simulink model "Microgrid"  (R2020b)
settings: Solver=VariableStepAuto  StartTime=0.0  StopTime=5  RelTol=1e-3
libraries: dspstat3 x1
settings Model: Creator=Stefano  LastModifiedBy=stefanopanzieri
settings SFSimCC: CustomCodeUndefinedFunction=UseInterfaceOnly

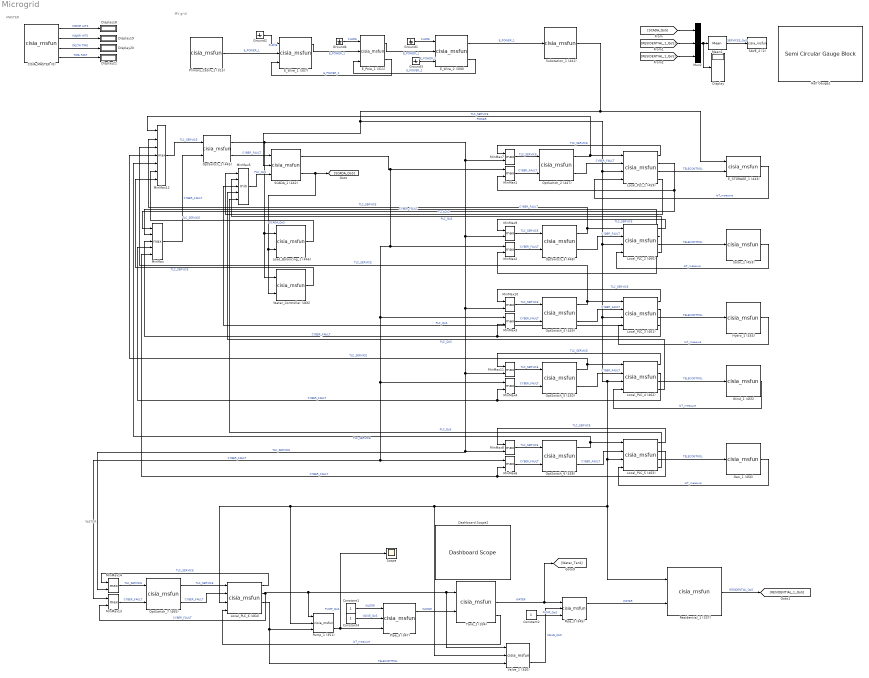
== system Microgrid ==
  note: MV grid
  note: MASTER
  note: WATER
  CISIA_MASTER (0) : M-S-Function  FunctionName=cisia_msfun  Parameters=Parameter1, Parameter2, Parameter3, resources, Parameter4, Parameter5, Parameter6, Parameter7, Parameter8, Parameter9  mask(S-function:msfcn_unit_delay){Parameter1='CISIA_MASTER', Parameter2=0.001, Parameter3='SistemiIoT', resources=off, Parameter4=on, Parameter5=off, Parameter6=off, Parameter7=off, Parameter8=1, Parameter9=off}
      mask prompts: Parameter1 "entity name"; Parameter2 "sampling time"; Parameter3 "project"; resources "Save status at each major hit"; Parameter4 "Show Operative Levels with colors"; Parameter5 "Load Entities from file"; Parameter6 "Load Start from Mask"; Parameter7 "Real Time"; Parameter8 "Real Time Hit (sec)"; Parameter9 "Skip saving"
      mask help: This is a level-2 MATLAB file S-function which demonstrates CISIA entity
      mask Display: disp('MASTER BLOCK')
  Constant1 : Constant
  Constant2 : Constant
  Constant4 : Constant
  Dashboard Scope2 : DashboardScope  Ymin=0  Ymax=1
  Display{,18..21} (5 alike) : Display
  E_Pole_1 (311) : M-S-Function  FunctionName=cisia_msfun  Parameters=Parameter1, Parameter2, Parameter3, resources, Parameter10, codeupdate, step_received, step_computed, dynamic_computed, step_sended, id_entity, id_project, id_type, name_type, color  mask(S-function:msfcn_unit_delay){Parameter1='E_Pole_1', Parameter2=1, Parameter3='', resources=|, Parameter10=off, codeupdate=off, step_received=|, step_computed=, dynamic_computed=, step_sended=|, id_entity=311, id_project=6, id_type=68, name_type=Electric_Pole, color=#FFFFFF}
      mask resources=|
      | *** INPUT RESOURCES ***
      | NUM_INPUTS 3
      | FLAME (1)
      | E_POWER_1 (10)
      | E_POWER_2 (10)
      |
      | *** STATE VARIABLES ***
      | NUM_VARIABLES 5
      | Operative_Level(NUMERIC)(1)(1)
      | Mechanical_Fault(NUMERIC)(1)(0)
      | Fire_Fault(NUMERIC)(1)(0)
      | Physical_Fault(NUMERIC)(1)(0)
      | Power_Gen(NUMERIC_ARRAY)(10)(0  0  0  0  0  0  0  0  0  0)
      |
      | *** OUTPUT RESOURCES ***
      | NUM_OUTPUTS 2
      | E_POWER_1 (10)
      | E_POWER_2 (10)
      mask step_received=|
      | Power_Gen=max(E_POWER_1,E_POWER_2);
      |
      | Fire_Fault=FLAME;
      |
      | Physical_Fault=max(Fire_Fault,Mechanical_Fault);
      |
      | Operative_Level=1-Physical_Fault;
      mask step_sended=|
      | E_POWER_1=Power_Gen*(1-Physical_Fault);
      | E_POWER_2=Power_Gen*(1-Physical_Fault);
      mask prompts: Parameter1 "entity name"; Parameter2 "sampling time"; Parameter3 "project"; resources "input resources and state variables"; Parameter10 "Bring state variables to output"; codeupdate "update code from mask"
      mask help: This is a level-2 MATLAB file S-function which demonstrates CISIA entity
      mask DialogControl Container1 Prompt: All parameters
      mask Display: image('Icons/Electric_Pole.png')
  E_STORAGE_1 (443) : M-S-Function  FunctionName=cisia_msfun  Parameters=Parameter1, Parameter2, Parameter3, resources, Parameter10, codeupdate, step_received, step_computed, dynamic_computed, step_sended, id_entity, id_project, id_type, name_type, color  mask(S-function:msfcn_unit_delay){Parameter1='E_STORAGE_1', Parameter2=1, Parameter3='', resources=|, Parameter10=off, codeupdate=off, step_received=|, step_computed=, dynamic_computed=, step_sended=IoT_measure=(1-IoT_Fault)*Operative_Level;, id_entity=443, id_project=6, id_type=101, name_type=Energy_Storage, color=#FFFFFF}
      mask resources=|
      | *** INPUT RESOURCES ***
      | NUM_INPUTS 2
      | POWER (1)
      | TELECONTROL (1)
      |
      | *** STATE VARIABLES ***
      | NUM_VARIABLES 5
      | Operative_Level(NUMERIC)(1)(1)
      | Cyber_Fault(NUMERIC_ARRAY)(10)(0  0  0  0  0  0  0  0  0  0)
      | Mechanical_Fault(NUMERIC)(1)(0)
      | Control_Fault(NUMERIC)(1)(0)
      | IoT_Fault(NUMERIC)(1)(0)
      |
      | *** OUTPUT RESOURCES ***
      | NUM_OUTPUTS 1
      | IoT_measure (1)
      mask step_received=|
      | Control_Fault=max([1-TELECONTROL Mechanical_Fault]);
      |
      | Operative_Level=min([1- Control_Fault 1-Mechanical_Fault POWER]);
      mask prompts: Parameter1 "entity name"; Parameter2 "sampling time"; Parameter3 "project"; resources "input resources and state variables"; Parameter10 "Bring state variables to output"; codeupdate "update code from mask"
      mask help: This is a level-2 MATLAB file S-function which demonstrates CISIA entity
      mask DialogControl Container1 Prompt: All parameters
      mask Display: image('Icons/Energy_Storage.png')
  E_Wire_1 (307) : M-S-Function  FunctionName=cisia_msfun  Parameters=Parameter1, Parameter2, Parameter3, resources, Parameter10, codeupdate, step_received, step_computed, dynamic_computed, step_sended, id_entity, id_project, id_type, name_type, color  mask(S-function:msfcn_unit_delay){Parameter1='E_Wire_1', Parameter2=1, Parameter3='', resources=|, Parameter10=off, codeupdate=off, step_received=|, step_computed=, dynamic_computed=, step_sended=|, id_entity=307, id_project=6, id_type=67, name_type=Electric_Wire, color=#FFFFFF}
      mask resources=|
      | *** INPUT RESOURCES ***
      | NUM_INPUTS 3
      | FLAME (1)
      | E_POWER_1 (10)
      | E_POWER_2 (10)
      |
      | *** STATE VARIABLES ***
      | NUM_VARIABLES 5
      | Operative_Level(NUMERIC)(1)(1)
      | Mechanical_Fault(NUMERIC)(1)(0)
      | Fire_Fault(NUMERIC)(1)(0)
      | Physical_Fault(NUMERIC)(1)(0)
      | Power_Gen(NUMERIC_ARRAY)(10)(0  0  0  0  0  0  0  0  0  0)
      |
      | *** OUTPUT RESOURCES ***
      | NUM_OUTPUTS 2
      | E_POWER_1 (10)
      | E_POWER_2 (10)
      mask step_received=|
      | Power_Gen=max(E_POWER_1,E_POWER_2);
      |
      | Fire_Fault=FLAME;
      |
      | Physical_Fault=max(Fire_Fault,Mechanical_Fault);
      |
      | Operative_Level=1-Physical_Fault;
      mask step_sended=|
      | E_POWER_1=Power_Gen*(1-Physical_Fault);
      | E_POWER_2=Power_Gen*(1-Physical_Fault);
      mask prompts: Parameter1 "entity name"; Parameter2 "sampling time"; Parameter3 "project"; resources "input resources and state variables"; Parameter10 "Bring state variables to output"; codeupdate "update code from mask"
      mask help: This is a level-2 MATLAB file S-function which demonstrates CISIA entity
      mask DialogControl Container1 Prompt: All parameters
      mask Display: image('Icons/Electric_Wire.png')
  E_Wire_2 (308) : M-S-Function  FunctionName=cisia_msfun  Parameters=Parameter1, Parameter2, Parameter3, resources, Parameter10, codeupdate, step_received, step_computed, dynamic_computed, step_sended, id_entity, id_project, id_type, name_type, color  mask(S-function:msfcn_unit_delay){Parameter1='E_Wire_2', Parameter2=1, Parameter3='', resources=|, Parameter10=off, codeupdate=off, step_received=|, step_computed=, dynamic_computed=, step_sended=|, id_entity=308, id_project=6, id_type=67, name_type=Electric_Wire, color=#FFFFFF}
      mask resources=|
      | *** INPUT RESOURCES ***
      | NUM_INPUTS 3
      | FLAME (1)
      | E_POWER_1 (10)
      | E_POWER_2 (10)
      |
      | *** STATE VARIABLES ***
      | NUM_VARIABLES 5
      | Operative_Level(NUMERIC)(1)(1)
      | Mechanical_Fault(NUMERIC)(1)(0)
      | Fire_Fault(NUMERIC)(1)(0)
      | Physical_Fault(NUMERIC)(1)(0)
      | Power_Gen(NUMERIC_ARRAY)(10)(0  0  0  0  0  0  0  0  0  0)
      |
      | *** OUTPUT RESOURCES ***
      | NUM_OUTPUTS 2
      | E_POWER_1 (10)
      | E_POWER_2 (10)
      mask step_received=|
      | Power_Gen=max(E_POWER_1,E_POWER_2);
      |
      | Fire_Fault=FLAME;
      |
      | Physical_Fault=max(Fire_Fault,Mechanical_Fault);
      |
      | Operative_Level=1-Physical_Fault;
      mask step_sended=|
      | E_POWER_1=Power_Gen*(1-Physical_Fault);
      | E_POWER_2=Power_Gen*(1-Physical_Fault);
      mask prompts: Parameter1 "entity name"; Parameter2 "sampling time"; Parameter3 "project"; resources "input resources and state variables"; Parameter10 "Bring state variables to output"; codeupdate "update code from mask"
      mask help: This is a level-2 MATLAB file S-function which demonstrates CISIA entity
      mask DialogControl Container1 Prompt: All parameters
      mask Display: image('Icons/Electric_Wire.png')
  Geo_1 (456) : M-S-Function  FunctionName=cisia_msfun  Parameters=Parameter1, Parameter2, Parameter3, resources, Parameter10, codeupdate, step_received, step_computed, dynamic_computed, step_sended, id_entity, id_project, id_type, name_type, color  mask(S-function:msfcn_unit_delay){Parameter1='Geo_1', Parameter2=1, Parameter3='', resources=|, Parameter10=off, codeupdate=off, step_received=|, step_computed=, dynamic_computed=, step_sended=IoT_measure=(1-IoT_Fault)*Operative_Level;, id_entity=456, id_project=6, id_type=107, name_type=Geothermic, color=#FFFFFF}
      mask resources=|
      | *** INPUT RESOURCES ***
      | NUM_INPUTS 1
      | TELECONTROL (1)
      |
      | *** STATE VARIABLES ***
      | NUM_VARIABLES 5
      | Operative_Level(NUMERIC)(1)(1)
      | Mechanical_Fault(NUMERIC)(1)(0)
      | Consumed_Services(NUMERIC_ARRAY)(20)(1  0  0  0  0  0  0  0  0  0  0  0  0  0  0  0  0  0  0  0)
      | Control_Fault(NUMERIC)(1)(0)
      | IoT_Fault(NUMERIC)(1)(0)
      |
      | *** OUTPUT RESOURCES ***
      | NUM_OUTPUTS 1
      | IoT_measure (1)
      mask step_received=|
      | Control_Fault=max([1-TELECONTROL Mechanical_Fault]);
      |
      | Operative_Level=min([1- Control_Fault 1-Mechanical_Fault]);
      mask prompts: Parameter1 "entity name"; Parameter2 "sampling time"; Parameter3 "project"; resources "input resources and state variables"; Parameter10 "Bring state variables to output"; codeupdate "update code from mask"
      mask help: This is a level-2 MATLAB file S-function which demonstrates CISIA entity
      mask DialogControl Container1 Prompt: All parameters
      mask Display: image('Icons/Geothermic.png')
  Ground{1..4} (4 alike) : Ground
  Half Gauge1 : SemiCircularGaugeBlock  ScaleMax=1
  Hydro_1 (454) : M-S-Function  FunctionName=cisia_msfun  Parameters=Parameter1, Parameter2, Parameter3, resources, Parameter10, codeupdate, step_received, step_computed, dynamic_computed, step_sended, id_entity, id_project, id_type, name_type, color  mask(S-function:msfcn_unit_delay){Parameter1='Hydro_1', Parameter2=1, Parameter3='', resources=|, Parameter10=off, codeupdate=off, step_received=|, step_computed=, dynamic_computed=, step_sended=IoT_measure=(1-IoT_Fault)*Operative_Level;, id_entity=454, id_project=6, id_type=105, name_type=Hydroelectric, color=#FFFFFF}
      mask resources=|
      | *** INPUT RESOURCES ***
      | NUM_INPUTS 1
      | TELECONTROL (1)
      |
      | *** STATE VARIABLES ***
      | NUM_VARIABLES 5
      | Operative_Level(NUMERIC)(1)(1)
      | Mechanical_Fault(NUMERIC)(1)(0)
      | Consumed_Services(NUMERIC_ARRAY)(20)(1  0  0  0  0  0  0  0  0  0  0  0  0  0  0  0  0  0  0  0)
      | Control_Fault(NUMERIC)(1)(0)
      | IoT_Fault(NUMERIC)(1)(0)
      |
      | *** OUTPUT RESOURCES ***
      | NUM_OUTPUTS 1
      | IoT_measure (1)
      mask step_received=|
      | Control_Fault=max([1-TELECONTROL Mechanical_Fault]);
      |
      | Operative_Level=min([1- Control_Fault 1-Mechanical_Fault]);
      mask prompts: Parameter1 "entity name"; Parameter2 "sampling time"; Parameter3 "project"; resources "input resources and state variables"; Parameter10 "Bring state variables to output"; codeupdate "update code from mask"
      mask help: This is a level-2 MATLAB file S-function which demonstrates CISIA entity
      mask DialogControl Container1 Prompt: All parameters
      mask Display: image('Icons/Hydroelectric.png')
  Load_Balancing_1 (446) : M-S-Function  FunctionName=cisia_msfun  Parameters=Parameter1, Parameter2, Parameter3, resources, Parameter10, codeupdate, step_received, step_computed, dynamic_computed, step_sended, id_entity, id_project, id_type, name_type, color  mask(S-function:msfcn_unit_delay){Parameter1='Load_Balancing_1', Parameter2=1, Parameter3='', resources=|, Parameter10=off, codeupdate=off, step_received=|, step_computed=, dynamic_computed=, step_sended=TLC_SERVICE=TLC_services*(1-Mechanical_Fault);, id_entity=446, id_project=6, id_type=103, name_type=Intelligent_Controller, color=#FFFFFF}
      mask resources=|
      | *** INPUT RESOURCES ***
      | NUM_INPUTS 2
      | TLC_SERVICE (20)
      | SCADA_QoS (1)
      |
      | *** STATE VARIABLES ***
      | NUM_VARIABLES 5
      | Operative_Level(NUMERIC)(1)(1)
      | TLC_services(NUMERIC_ARRAY)(20)(1  0  0  0  0  0  0  0  0  0  0  0  0  0  0  0  0  0  0  0)
      | Mechanical_Fault(NUMERIC)(1)(0)
      | Consumed_Services(NUMERIC_ARRAY)(20)(0  1  1  1  1  1  0  0  0  0  0  0  0  0  0  0  0  0  0  0)
      | Service_Fault(NUMERIC)(1)(0)
      |
      | *** OUTPUT RESOURCES ***
      | NUM_OUTPUTS 1
      | TLC_SERVICE (20)
      mask step_received=|
      | TLC_services=max(TLC_services_init,TLC_SERVICE);
      |
      | Service_Fault=max(abs(Consumed_Services.*TLC_services-Consumed_Services));
      |
      | Operative_Level=min([1-Mechanical_Fault 1-Service_Fault]);
      mask prompts: Parameter1 "entity name"; Parameter2 "sampling time"; Parameter3 "project"; resources "input resources and state variables"; Parameter10 "Bring state variables to output"; codeupdate "update code from mask"
      mask help: This is a level-2 MATLAB file S-function which demonstrates CISIA entity
      mask DialogControl Container1 Prompt: All parameters
      mask Display: image('Icons/Intelligent_Controller.png')
  Local_PLC_1 (459) : M-S-Function  FunctionName=cisia_msfun  Parameters=Parameter1, Parameter2, Parameter3, resources, Parameter10, codeupdate, step_received, step_computed, dynamic_computed, step_sended, id_entity, id_project, id_type, name_type, color  mask(S-function:msfcn_unit_delay){Parameter1='Local_PLC_1', Parameter2=1, Parameter3='', resources=|, Parameter10=off, codeupdate=off, step_received=|, step_computed=, dynamic_computed=, step_sended=|, id_entity=459, id_project=6, id_type=108, name_type=LocalController, color=#FFFFFF}
      mask resources=|
      | *** INPUT RESOURCES ***
      | NUM_INPUTS 4
      | TLC_SERVICE (20)
      | CYBER_FAULT (10)
      | POWER (1)
      | IoT_measure (1)
      |
      | *** STATE VARIABLES ***
      | NUM_VARIABLES 17
      | Operative_Level(NUMERIC)(1)(1)
      | TLC_services(NUMERIC_ARRAY)(20)(0  1  0  0  0  0  0  0  0  0  0  0  0  0  0  0  0  0  0  0)
      | Dos_attack(NUMERIC)(1)(0)
      | MITM_attack(NUMERIC)(1)(0)
      | Virus_Attack(NUMERIC)(1)(0)
      | Port_Scan_Attack(NUMERIC)(1)(0)
      | Cyber_Fault(NUMERIC_ARRAY)(10)(0  0  0  0  0  0  0  0  0  0)
      | BGP_hijacking(NUMERIC)(1)(0)
      | Mechanical_Fault(NUMERIC)(1)(0)
      | Consumed_Services(NUMERIC_ARRAY)(20)(1  0  0  0  0  0  0  0  0  0  0  0  0  0  0  0  0  0  0  0)
      | Service_Fault(NUMERIC)(1)(0)
      | BotNet_Attack(NUMERIC)(1)(0)
      | Data_Corruption(NUMERIC)(1)(0)
      | SW_Change(NUMERIC)(1)(0)
      | Config_Change(NUMERIC)(1)(0)
      | Port_Saturation(NUMERIC)(1)(0)
      | Control_Fault(NUMERIC)(1)(0)
      |
      | *** OUTPUT RESOURCES ***
      | NUM_OUTPUTS 4
      | TLC_SERVICE (20)
      | CYBER_FAULT (10)
      | TELECONTROL (1)
      | PLC_QoS (1)
      mask step_received=|
      | TLC_services=max(TLC_services_init,TLC_SERVICE);
      |
      | Service_Fault=max(abs(Consumed_Services.*TLC_services-Consumed_Services));
      |
      | Cyber_Fault=max(CYBER_FAULT, transpose([Dos_attack MITM_attack Virus_Attack Port_Scan_Attack  BGP_hijacking BotNet_Attack Data_Corruption SW_Change Config_Change Port_Saturation]));
      |
      |
      | %Control_Fault=max([1-Service_Fault Mechanical_Fault 1-POWER Dos_attack min(0.5,max(Cyber_Fault))]);
      |
      | Control_Fault=max([Service_Fault Mechanical_Fault 1-POWER Dos_attack min(0.5,max(Cyber_Fault))]);
      |
      |
      | Operative_Level=min([1-max(Cyber_Fault) 1-Mechanical_Fault 1-Control_Fault 1-Service_Fault]);
      mask step_sended=|
      | CYBER_FAULT=Cyber_Fault.*transpose([0 0 0.5 0.2 0 0 0 0 0 0]);
      |
      | TELECONTROL=1-Control_Fault;
      | PLC_QoS=Operative_Level;
      |
      | TLC_SERVICE=TLC_services;
      mask prompts: Parameter1 "entity name"; Parameter2 "sampling time"; Parameter3 "project"; resources "input resources and state variables"; Parameter10 "Bring state variables to output"; codeupdate "update code from mask"
      mask help: This is a level-2 MATLAB file S-function which demonstrates CISIA entity
      mask DialogControl Container1 Prompt: All parameters
      mask Display: image('Icons/LocalController.png')
  Local_PLC_2 (460) : M-S-Function  FunctionName=cisia_msfun  Parameters=Parameter1, Parameter2, Parameter3, resources, Parameter10, codeupdate, step_received, step_computed, dynamic_computed, step_sended, id_entity, id_project, id_type, name_type, color  mask(S-function:msfcn_unit_delay){Parameter1='Local_PLC_2', Parameter2=1, Parameter3='', resources=|, Parameter10=off, codeupdate=off, step_received=|, step_computed=, dynamic_computed=, step_sended=|, id_entity=460, id_project=6, id_type=108, name_type=LocalController, color=#FFFFFF}
      mask resources=|
      | *** INPUT RESOURCES ***
      | NUM_INPUTS 4
      | TLC_SERVICE (20)
      | CYBER_FAULT (10)
      | POWER (1)
      | IoT_measure (1)
      |
      | *** STATE VARIABLES ***
      | NUM_VARIABLES 17
      | Operative_Level(NUMERIC)(1)(0)
      | TLC_services(NUMERIC_ARRAY)(20)(0  0  1  0  0  0  0  0  0  0  0  0  0  0  0  0  0  0  0  0)
      | Dos_attack(NUMERIC)(1)(0.5)
      | MITM_attack(NUMERIC)(1)(0)
      | Virus_Attack(NUMERIC)(1)(0)
      | Port_Scan_Attack(NUMERIC)(1)(0)
      | Cyber_Fault(NUMERIC_ARRAY)(10)(0  0  0  0  0  0  0  0  0  0)
      | BGP_hijacking(NUMERIC)(1)(0)
      | Mechanical_Fault(NUMERIC)(1)(0)
      | Consumed_Services(NUMERIC_ARRAY)(20)(1  0  0  0  0  0  0  0  0  0  0  0  0  0  0  0  0  0  0  0)
      | Service_Fault(NUMERIC)(1)(0)
      | BotNet_Attack(NUMERIC)(1)(0)
      | Data_Corruption(NUMERIC)(1)(0)
      | SW_Change(NUMERIC)(1)(0)
      | Config_Change(NUMERIC)(1)(0)
      | Port_Saturation(NUMERIC)(1)(0)
      | Control_Fault(NUMERIC)(1)(0)
      |
      | *** OUTPUT RESOURCES ***
      | NUM_OUTPUTS 4
      | TLC_SERVICE (20)
      | CYBER_FAULT (10)
      | TELECONTROL (1)
      | PLC_QoS (1)
      mask step_received=|
      | TLC_services=max(TLC_services_init,TLC_SERVICE);
      |
      | Service_Fault=max(abs(Consumed_Services.*TLC_services-Consumed_Services));
      |
      | Cyber_Fault=max(CYBER_FAULT, transpose([Dos_attack MITM_attack Virus_Attack Port_Scan_Attack  BGP_hijacking BotNet_Attack Data_Corruption SW_Change Config_Change Port_Saturation]));
      |
      |
      | %Control_Fault=max([1-Service_Fault Mechanical_Fault 1-POWER Dos_attack min(0.5,max(Cyber_Fault))]);
      |
      | Control_Fault=max([Service_Fault Mechanical_Fault 1-POWER Dos_attack min(0.5,max(Cyber_Fault))]);
      |
      |
      | Operative_Level=min([1-max(Cyber_Fault) 1-Mechanical_Fault 1-Control_Fault 1-Service_Fault]);
      mask step_sended=|
      | CYBER_FAULT=Cyber_Fault.*transpose([0 0 0.5 0.2 0 0 0 0 0 0]);
      |
      | TELECONTROL=1-Control_Fault;
      | PLC_QoS=Operative_Level;
      |
      | TLC_SERVICE=TLC_services;
      mask prompts: Parameter1 "entity name"; Parameter2 "sampling time"; Parameter3 "project"; resources "input resources and state variables"; Parameter10 "Bring state variables to output"; codeupdate "update code from mask"
      mask help: This is a level-2 MATLAB file S-function which demonstrates CISIA entity
      mask DialogControl Container1 Prompt: All parameters
      mask Display: image('Icons/LocalController.png')
  Local_PLC_3 (461) : M-S-Function  FunctionName=cisia_msfun  Parameters=Parameter1, Parameter2, Parameter3, resources, Parameter10, codeupdate, step_received, step_computed, dynamic_computed, step_sended, id_entity, id_project, id_type, name_type, color  mask(S-function:msfcn_unit_delay){Parameter1='Local_PLC_3', Parameter2=1, Parameter3='', resources=|, Parameter10=off, codeupdate=off, step_received=|, step_computed=, dynamic_computed=, step_sended=|, id_entity=461, id_project=6, id_type=108, name_type=LocalController, color=#FFFFFF}
      mask resources=|
      | *** INPUT RESOURCES ***
      | NUM_INPUTS 4
      | TLC_SERVICE (20)
      | CYBER_FAULT (10)
      | POWER (1)
      | IoT_measure (1)
      |
      | *** STATE VARIABLES ***
      | NUM_VARIABLES 17
      | Operative_Level(NUMERIC)(1)(0)
      | TLC_services(NUMERIC_ARRAY)(20)(0  0  0  1  0  0  0  0  0  0  0  0  0  0  0  0  0  0  0  0)
      | Dos_attack(NUMERIC)(1)(0)
      | MITM_attack(NUMERIC)(1)(0)
      | Virus_Attack(NUMERIC)(1)(0)
      | Port_Scan_Attack(NUMERIC)(1)(0)
      | Cyber_Fault(NUMERIC_ARRAY)(10)(0  0  0  0  0  0  0  0  0  0)
      | BGP_hijacking(NUMERIC)(1)(0)
      | Mechanical_Fault(NUMERIC)(1)(0)
      | Consumed_Services(NUMERIC_ARRAY)(20)(1  0  0  0  0  0  0  0  0  0  0  0  0  0  0  0  0  0  0  0)
      | Service_Fault(NUMERIC)(1)(0)
      | BotNet_Attack(NUMERIC)(1)(0)
      | Data_Corruption(NUMERIC)(1)(0)
      | SW_Change(NUMERIC)(1)(0)
      | Config_Change(NUMERIC)(1)(0)
      | Port_Saturation(NUMERIC)(1)(0)
      | Control_Fault(NUMERIC)(1)(0)
      |
      | *** OUTPUT RESOURCES ***
      | NUM_OUTPUTS 4
      | TLC_SERVICE (20)
      | CYBER_FAULT (10)
      | TELECONTROL (1)
      | PLC_QoS (1)
      mask step_received=|
      | TLC_services=max(TLC_services_init,TLC_SERVICE);
      |
      | Service_Fault=max(abs(Consumed_Services.*TLC_services-Consumed_Services));
      |
      | Cyber_Fault=max(CYBER_FAULT, transpose([Dos_attack MITM_attack Virus_Attack Port_Scan_Attack  BGP_hijacking BotNet_Attack Data_Corruption SW_Change Config_Change Port_Saturation]));
      |
      |
      | %Control_Fault=max([1-Service_Fault Mechanical_Fault 1-POWER Dos_attack min(0.5,max(Cyber_Fault))]);
      |
      | Control_Fault=max([Service_Fault Mechanical_Fault 1-POWER Dos_attack min(0.5,max(Cyber_Fault))]);
      |
      |
      | Operative_Level=min([1-max(Cyber_Fault) 1-Mechanical_Fault 1-Control_Fault 1-Service_Fault]);
      mask step_sended=|
      | CYBER_FAULT=Cyber_Fault.*transpose([0 0 0.5 0.2 0 0 0 0 0 0]);
      |
      | TELECONTROL=1-Control_Fault;
      | PLC_QoS=Operative_Level;
      |
      | TLC_SERVICE=TLC_services;
      mask prompts: Parameter1 "entity name"; Parameter2 "sampling time"; Parameter3 "project"; resources "input resources and state variables"; Parameter10 "Bring state variables to output"; codeupdate "update code from mask"
      mask help: This is a level-2 MATLAB file S-function which demonstrates CISIA entity
      mask DialogControl Container1 Prompt: All parameters
      mask Display: image('Icons/LocalController.png')
  Local_PLC_4 (462) : M-S-Function  FunctionName=cisia_msfun  Parameters=Parameter1, Parameter2, Parameter3, resources, Parameter10, codeupdate, step_received, step_computed, dynamic_computed, step_sended, id_entity, id_project, id_type, name_type, color  mask(S-function:msfcn_unit_delay){Parameter1='Local_PLC_4', Parameter2=1, Parameter3='', resources=|, Parameter10=off, codeupdate=off, step_received=|, step_computed=, dynamic_computed=, step_sended=|, id_entity=462, id_project=6, id_type=108, name_type=LocalController, color=#FFFFFF}
      mask resources=|
      | *** INPUT RESOURCES ***
      | NUM_INPUTS 4
      | TLC_SERVICE (20)
      | CYBER_FAULT (10)
      | POWER (1)
      | IoT_measure (1)
      |
      | *** STATE VARIABLES ***
      | NUM_VARIABLES 17
      | Operative_Level(NUMERIC)(1)(0)
      | TLC_services(NUMERIC_ARRAY)(20)(0  0  0  0  1  0  0  0  0  0  0  0  0  0  0  0  0  0  0  0)
      | Dos_attack(NUMERIC)(1)(0)
      | MITM_attack(NUMERIC)(1)(0)
      | Virus_Attack(NUMERIC)(1)(0)
      | Port_Scan_Attack(NUMERIC)(1)(0)
      | Cyber_Fault(NUMERIC_ARRAY)(10)(0  0  0  0  0  0  0  0  0  0)
      | BGP_hijacking(NUMERIC)(1)(0)
      | Mechanical_Fault(NUMERIC)(1)(0)
      | Consumed_Services(NUMERIC_ARRAY)(20)(1  0  0  0  0  0  0  0  0  0  0  0  0  0  0  0  0  0  0  0)
      | Service_Fault(NUMERIC)(1)(0)
      | BotNet_Attack(NUMERIC)(1)(0)
      | Data_Corruption(NUMERIC)(1)(0)
      | SW_Change(NUMERIC)(1)(0)
      | Config_Change(NUMERIC)(1)(0)
      | Port_Saturation(NUMERIC)(1)(0)
      | Control_Fault(NUMERIC)(1)(0)
      |
      | *** OUTPUT RESOURCES ***
      | NUM_OUTPUTS 4
      | TLC_SERVICE (20)
      | CYBER_FAULT (10)
      | TELECONTROL (1)
      | PLC_QoS (1)
      mask step_received=|
      | TLC_services=max(TLC_services_init,TLC_SERVICE);
      |
      | Service_Fault=max(abs(Consumed_Services.*TLC_services-Consumed_Services));
      |
      | Cyber_Fault=max(CYBER_FAULT, transpose([Dos_attack MITM_attack Virus_Attack Port_Scan_Attack  BGP_hijacking BotNet_Attack Data_Corruption SW_Change Config_Change Port_Saturation]));
      |
      |
      | %Control_Fault=max([1-Service_Fault Mechanical_Fault 1-POWER Dos_attack min(0.5,max(Cyber_Fault))]);
      |
      | Control_Fault=max([Service_Fault Mechanical_Fault 1-POWER Dos_attack min(0.5,max(Cyber_Fault))]);
      |
      |
      | Operative_Level=min([1-max(Cyber_Fault) 1-Mechanical_Fault 1-Control_Fault 1-Service_Fault]);
      mask step_sended=|
      | CYBER_FAULT=Cyber_Fault.*transpose([0 0 0.5 0.2 0 0 0 0 0 0]);
      |
      | TELECONTROL=1-Control_Fault;
      | PLC_QoS=Operative_Level;
      |
      | TLC_SERVICE=TLC_services;
      mask prompts: Parameter1 "entity name"; Parameter2 "sampling time"; Parameter3 "project"; resources "input resources and state variables"; Parameter10 "Bring state variables to output"; codeupdate "update code from mask"
      mask help: This is a level-2 MATLAB file S-function which demonstrates CISIA entity
      mask DialogControl Container1 Prompt: All parameters
      mask Display: image('Icons/LocalController.png')
  Local_PLC_5 (463) : M-S-Function  FunctionName=cisia_msfun  Parameters=Parameter1, Parameter2, Parameter3, resources, Parameter10, codeupdate, step_received, step_computed, dynamic_computed, step_sended, id_entity, id_project, id_type, name_type, color  mask(S-function:msfcn_unit_delay){Parameter1='Local_PLC_5', Parameter2=1, Parameter3='', resources=|, Parameter10=off, codeupdate=off, step_received=|, step_computed=, dynamic_computed=, step_sended=|, id_entity=463, id_project=6, id_type=108, name_type=LocalController, color=#FFFFFF}
      mask resources=|
      | *** INPUT RESOURCES ***
      | NUM_INPUTS 4
      | TLC_SERVICE (20)
      | CYBER_FAULT (10)
      | POWER (1)
      | IoT_measure (1)
      |
      | *** STATE VARIABLES ***
      | NUM_VARIABLES 17
      | Operative_Level(NUMERIC)(1)(0)
      | TLC_services(NUMERIC_ARRAY)(20)(0  0  0  0  0  1  0  0  0  0  0  0  0  0  0  0  0  0  0  0)
      | Dos_attack(NUMERIC)(1)(0)
      | MITM_attack(NUMERIC)(1)(0)
      | Virus_Attack(NUMERIC)(1)(0)
      | Port_Scan_Attack(NUMERIC)(1)(0)
      | Cyber_Fault(NUMERIC_ARRAY)(10)(0  0  0  0  0  0  0  0  0  0)
      | BGP_hijacking(NUMERIC)(1)(0)
      | Mechanical_Fault(NUMERIC)(1)(0)
      | Consumed_Services(NUMERIC_ARRAY)(20)(1  0  0  0  0  0  0  0  0  0  0  0  0  0  0  0  0  0  0  0)
      | Service_Fault(NUMERIC)(1)(0)
      | BotNet_Attack(NUMERIC)(1)(0)
      | Data_Corruption(NUMERIC)(1)(0)
      | SW_Change(NUMERIC)(1)(0)
      | Config_Change(NUMERIC)(1)(0)
      | Port_Saturation(NUMERIC)(1)(0)
      | Control_Fault(NUMERIC)(1)(0)
      |
      | *** OUTPUT RESOURCES ***
      | NUM_OUTPUTS 4
      | TLC_SERVICE (20)
      | CYBER_FAULT (10)
      | TELECONTROL (1)
      | PLC_QoS (1)
      mask step_received=|
      | TLC_services=max(TLC_services_init,TLC_SERVICE);
      |
      | Service_Fault=max(abs(Consumed_Services.*TLC_services-Consumed_Services));
      |
      | Cyber_Fault=max(CYBER_FAULT, transpose([Dos_attack MITM_attack Virus_Attack Port_Scan_Attack  BGP_hijacking BotNet_Attack Data_Corruption SW_Change Config_Change Port_Saturation]));
      |
      |
      | %Control_Fault=max([1-Service_Fault Mechanical_Fault 1-POWER Dos_attack min(0.5,max(Cyber_Fault))]);
      |
      | Control_Fault=max([Service_Fault Mechanical_Fault 1-POWER Dos_attack min(0.5,max(Cyber_Fault))]);
      |
      |
      | Operative_Level=min([1-max(Cyber_Fault) 1-Mechanical_Fault 1-Control_Fault 1-Service_Fault]);
      mask step_sended=|
      | CYBER_FAULT=Cyber_Fault.*transpose([0 0 0.5 0.2 0 0 0 0 0 0]);
      |
      | TELECONTROL=1-Control_Fault;
      | PLC_QoS=Operative_Level;
      |
      | TLC_SERVICE=TLC_services;
      mask prompts: Parameter1 "entity name"; Parameter2 "sampling time"; Parameter3 "project"; resources "input resources and state variables"; Parameter10 "Bring state variables to output"; codeupdate "update code from mask"
      mask help: This is a level-2 MATLAB file S-function which demonstrates CISIA entity
      mask DialogControl Container1 Prompt: All parameters
      mask Display: image('Icons/LocalController.png')
  Local_PLC_6 (464) : M-S-Function  FunctionName=cisia_msfun  Parameters=Parameter1, Parameter2, Parameter3, resources, Parameter10, codeupdate, step_received, step_computed, dynamic_computed, step_sended, id_entity, id_project, id_type, name_type, color  mask(S-function:msfcn_unit_delay){Parameter1='Local_PLC_6', Parameter2=1, Parameter3='', resources=|, Parameter10=off, codeupdate=off, step_received=|, step_computed=, dynamic_computed=, step_sended=|, id_entity=464, id_project=6, id_type=108, name_type=LocalController, color=#FFFFFF}
      mask resources=|
      | *** INPUT RESOURCES ***
      | NUM_INPUTS 4
      | TLC_SERVICE (20)
      | CYBER_FAULT (10)
      | POWER (1)
      | IoT_measure (1)
      |
      | *** STATE VARIABLES ***
      | NUM_VARIABLES 17
      | Operative_Level(NUMERIC)(1)(0)
      | TLC_services(NUMERIC_ARRAY)(20)(0  0  0  0  0  0  0  0  0  0  0  0  0  0  0  0  0  0  0  0)
      | Dos_attack(NUMERIC)(1)(0)
      | MITM_attack(NUMERIC)(1)(0)
      | Virus_Attack(NUMERIC)(1)(0)
      | Port_Scan_Attack(NUMERIC)(1)(0)
      | Cyber_Fault(NUMERIC_ARRAY)(10)(0  0  0  0  0  0  0  0  0  0)
      | BGP_hijacking(NUMERIC)(1)(0)
      | Mechanical_Fault(NUMERIC)(1)(0)
      | Consumed_Services(NUMERIC_ARRAY)(20)(0  0  0  0  0  0  1  0  0  0  0  0  0  0  0  0  0  0  0  0)
      | Service_Fault(NUMERIC)(1)(0)
      | BotNet_Attack(NUMERIC)(1)(0)
      | Data_Corruption(NUMERIC)(1)(0)
      | SW_Change(NUMERIC)(1)(0)
      | Config_Change(NUMERIC)(1)(0)
      | Port_Saturation(NUMERIC)(1)(0)
      | Control_Fault(NUMERIC)(1)(0)
      |
      | *** OUTPUT RESOURCES ***
      | NUM_OUTPUTS 4
      | TLC_SERVICE (20)
      | CYBER_FAULT (10)
      | TELECONTROL (1)
      | PLC_QoS (1)
      mask step_received=|
      | TLC_services=max(TLC_services_init,TLC_SERVICE);
      |
      | Service_Fault=max(abs(Consumed_Services.*TLC_services-Consumed_Services));
      |
      | Cyber_Fault=max(CYBER_FAULT, transpose([Dos_attack MITM_attack Virus_Attack Port_Scan_Attack  BGP_hijacking BotNet_Attack Data_Corruption SW_Change Config_Change Port_Saturation]));
      |
      |
      | %Control_Fault=max([1-Service_Fault Mechanical_Fault 1-POWER Dos_attack min(0.5,max(Cyber_Fault))]);
      |
      | Control_Fault=max([Service_Fault Mechanical_Fault 1-POWER Dos_attack min(0.5,max(Cyber_Fault))]);
      |
      |
      | Operative_Level=min([1-max(Cyber_Fault) 1-Mechanical_Fault 1-Control_Fault 1-Service_Fault]);
      mask step_sended=|
      | CYBER_FAULT=Cyber_Fault.*transpose([0 0 0.5 0.2 0 0 0 0 0 0]);
      |
      | TELECONTROL=1-Control_Fault;
      | PLC_QoS=Operative_Level;
      |
      | TLC_SERVICE=TLC_services;
      mask prompts: Parameter1 "entity name"; Parameter2 "sampling time"; Parameter3 "project"; resources "input resources and state variables"; Parameter10 "Bring state variables to output"; codeupdate "update code from mask"
      mask help: This is a level-2 MATLAB file S-function which demonstrates CISIA entity
      mask DialogControl Container1 Prompt: All parameters
      mask Display: image('Icons/LocalController.png')
  Mean1 : dspstat3/Mean  run=off  InputProcessing=Columns as channels (frame based)  reset_popup=None  directionMode=Each column  dimension=1  roiEnable=off  roiType=Rectangles  roiPortion=Entire ROI  roiOutput=Individual statistics for each ROI  roiFlag=off  roundingMode=Floor  overflowMode=off  outputDataTypeStr=Inherit: Same as accumulator  outputMin=[]  outputMax=[]  outputLastDataTypeStr=Inherit: Same as accumulator
  MinMax : MinMax  Function=max  Inputs=5
  MinMax{1..4,6..11,13..14} (12 alike) : MinMax  Function=max  Inputs=2
  MinMax12 : MinMax  Function=max  Inputs=7
  MinMax5 : MinMax  Inputs=5
  Mux2 : Mux  Inputs=3
  OptSwitch_1 (445) : M-S-Function  FunctionName=cisia_msfun  Parameters=Parameter1, Parameter2, Parameter3, resources, Parameter10, codeupdate, step_received, step_computed, dynamic_computed, step_sended, id_entity, id_project, id_type, name_type, color  mask(S-function:msfcn_unit_delay){Parameter1='OptSwitch_1', Parameter2=1, Parameter3='', resources=|, Parameter10=off, codeupdate=off, step_received=|, step_computed=, dynamic_computed=, step_sended=|, id_entity=445, id_project=6, id_type=102, name_type=Optical_Switch, color=#FFFFFF}
      mask resources=|
      | *** INPUT RESOURCES ***
      | NUM_INPUTS 2
      | TLC_SERVICE (20)
      | CYBER_FAULT (10)
      |
      | *** STATE VARIABLES ***
      | NUM_VARIABLES 4
      | Operative_Level(NUMERIC)(1)(1)
      | TLC_services(NUMERIC_ARRAY)(20)(0  0  0  0  0  0  0  0  0  0  0  0  0  0  0  0  0  0  0  0)
      | Cyber_Fault(NUMERIC_ARRAY)(10)(0  0  0  0  0  0  0  0  0  0)
      | Mechanical_Fault(NUMERIC)(1)(0)
      |
      | *** OUTPUT RESOURCES ***
      | NUM_OUTPUTS 2
      | TLC_SERVICE (20)
      | CYBER_FAULT (10)
      mask step_received=|
      | TLC_services=max(TLC_services_init,TLC_SERVICE);
      | Cyber_Fault=CYBER_FAULT;
      |
      | Operative_Level=min([1-Mechanical_Fault]);
      mask step_sended=|
      | CYBER_FAULT=Cyber_Fault;
      | TLC_SERVICE=TLC_services*Operative_Level;
      mask prompts: Parameter1 "entity name"; Parameter2 "sampling time"; Parameter3 "project"; resources "input resources and state variables"; Parameter10 "Bring state variables to output"; codeupdate "update code from mask"
      mask help: This is a level-2 MATLAB file S-function which demonstrates CISIA entity
      mask DialogControl Container1 Prompt: All parameters
      mask Display: image('Icons/Optical_Switch.png')
  OptSwitch_2 (447) : M-S-Function  FunctionName=cisia_msfun  Parameters=Parameter1, Parameter2, Parameter3, resources, Parameter10, codeupdate, step_received, step_computed, dynamic_computed, step_sended, id_entity, id_project, id_type, name_type, color  mask(S-function:msfcn_unit_delay){Parameter1='OptSwitch_2', Parameter2=1, Parameter3='', resources=|, Parameter10=off, codeupdate=off, step_received=|, step_computed=, dynamic_computed=, step_sended=|, id_entity=447, id_project=6, id_type=102, name_type=Optical_Switch, color=#FFFFFF}
      mask resources=|
      | *** INPUT RESOURCES ***
      | NUM_INPUTS 2
      | TLC_SERVICE (20)
      | CYBER_FAULT (10)
      |
      | *** STATE VARIABLES ***
      | NUM_VARIABLES 4
      | Operative_Level(NUMERIC)(1)(0)
      | TLC_services(NUMERIC_ARRAY)(20)(0  0  0  0  0  0  0  0  0  0  0  0  0  0  0  0  0  0  0  0)
      | Cyber_Fault(NUMERIC_ARRAY)(10)(0  0  0  0  0  0  0  0  0  0)
      | Mechanical_Fault(NUMERIC)(1)(0)
      |
      | *** OUTPUT RESOURCES ***
      | NUM_OUTPUTS 2
      | TLC_SERVICE (20)
      | CYBER_FAULT (10)
      mask step_received=|
      | TLC_services=max(TLC_services_init,TLC_SERVICE);
      | Cyber_Fault=CYBER_FAULT;
      |
      | Operative_Level=min([1-Mechanical_Fault]);
      mask step_sended=|
      | CYBER_FAULT=Cyber_Fault;
      | TLC_SERVICE=TLC_services*Operative_Level;
      mask prompts: Parameter1 "entity name"; Parameter2 "sampling time"; Parameter3 "project"; resources "input resources and state variables"; Parameter10 "Bring state variables to output"; codeupdate "update code from mask"
      mask help: This is a level-2 MATLAB file S-function which demonstrates CISIA entity
      mask DialogControl Container1 Prompt: All parameters
      mask Display: image('Icons/Optical_Switch.png')
  OptSwitch_3 (448) : M-S-Function  FunctionName=cisia_msfun  Parameters=Parameter1, Parameter2, Parameter3, resources, Parameter10, codeupdate, step_received, step_computed, dynamic_computed, step_sended, id_entity, id_project, id_type, name_type, color  mask(S-function:msfcn_unit_delay){Parameter1='OptSwitch_3', Parameter2=1, Parameter3='', resources=|, Parameter10=off, codeupdate=off, step_received=|, step_computed=, dynamic_computed=, step_sended=|, id_entity=448, id_project=6, id_type=102, name_type=Optical_Switch, color=#FFFFFF}
      mask resources=|
      | *** INPUT RESOURCES ***
      | NUM_INPUTS 2
      | TLC_SERVICE (20)
      | CYBER_FAULT (10)
      |
      | *** STATE VARIABLES ***
      | NUM_VARIABLES 4
      | Operative_Level(NUMERIC)(1)(0)
      | TLC_services(NUMERIC_ARRAY)(20)(0  0  0  0  0  0  0  0  0  0  0  0  0  0  0  0  0  0  0  0)
      | Cyber_Fault(NUMERIC_ARRAY)(10)(0  0  0  0  0  0  0  0  0  0)
      | Mechanical_Fault(NUMERIC)(1)(0)
      |
      | *** OUTPUT RESOURCES ***
      | NUM_OUTPUTS 2
      | TLC_SERVICE (20)
      | CYBER_FAULT (10)
      mask step_received=|
      | TLC_services=max(TLC_services_init,TLC_SERVICE);
      | Cyber_Fault=CYBER_FAULT;
      |
      | Operative_Level=min([1-Mechanical_Fault]);
      mask step_sended=|
      | CYBER_FAULT=Cyber_Fault;
      | TLC_SERVICE=TLC_services*Operative_Level;
      mask prompts: Parameter1 "entity name"; Parameter2 "sampling time"; Parameter3 "project"; resources "input resources and state variables"; Parameter10 "Bring state variables to output"; codeupdate "update code from mask"
      mask help: This is a level-2 MATLAB file S-function which demonstrates CISIA entity
      mask DialogControl Container1 Prompt: All parameters
      mask Display: image('Icons/Optical_Switch.png')
  OptSwitch_4 (449) : M-S-Function  FunctionName=cisia_msfun  Parameters=Parameter1, Parameter2, Parameter3, resources, Parameter10, codeupdate, step_received, step_computed, dynamic_computed, step_sended, id_entity, id_project, id_type, name_type, color  mask(S-function:msfcn_unit_delay){Parameter1='OptSwitch_4', Parameter2=1, Parameter3='', resources=|, Parameter10=off, codeupdate=off, step_received=|, step_computed=, dynamic_computed=, step_sended=|, id_entity=449, id_project=6, id_type=102, name_type=Optical_Switch, color=#FFFFFF}
      mask resources=|
      | *** INPUT RESOURCES ***
      | NUM_INPUTS 2
      | TLC_SERVICE (20)
      | CYBER_FAULT (10)
      |
      | *** STATE VARIABLES ***
      | NUM_VARIABLES 4
      | Operative_Level(NUMERIC)(1)(0)
      | TLC_services(NUMERIC_ARRAY)(20)(0  0  0  0  0  0  0  0  0  0  0  0  0  0  0  0  0  0  0  0)
      | Cyber_Fault(NUMERIC_ARRAY)(10)(0  0  0  0  0  0  0  0  0  0)
      | Mechanical_Fault(NUMERIC)(1)(0)
      |
      | *** OUTPUT RESOURCES ***
      | NUM_OUTPUTS 2
      | TLC_SERVICE (20)
      | CYBER_FAULT (10)
      mask step_received=|
      | TLC_services=max(TLC_services_init,TLC_SERVICE);
      | Cyber_Fault=CYBER_FAULT;
      |
      | Operative_Level=min([1-Mechanical_Fault]);
      mask step_sended=|
      | CYBER_FAULT=Cyber_Fault;
      | TLC_SERVICE=TLC_services*Operative_Level;
      mask prompts: Parameter1 "entity name"; Parameter2 "sampling time"; Parameter3 "project"; resources "input resources and state variables"; Parameter10 "Bring state variables to output"; codeupdate "update code from mask"
      mask help: This is a level-2 MATLAB file S-function which demonstrates CISIA entity
      mask DialogControl Container1 Prompt: All parameters
      mask Display: image('Icons/Optical_Switch.png')
  OptSwitch_5 (450) : M-S-Function  FunctionName=cisia_msfun  Parameters=Parameter1, Parameter2, Parameter3, resources, Parameter10, codeupdate, step_received, step_computed, dynamic_computed, step_sended, id_entity, id_project, id_type, name_type, color  mask(S-function:msfcn_unit_delay){Parameter1='OptSwitch_5', Parameter2=1, Parameter3='', resources=|, Parameter10=off, codeupdate=off, step_received=|, step_computed=, dynamic_computed=, step_sended=|, id_entity=450, id_project=6, id_type=102, name_type=Optical_Switch, color=#FFFFFF}
      mask resources=|
      | *** INPUT RESOURCES ***
      | NUM_INPUTS 2
      | TLC_SERVICE (20)
      | CYBER_FAULT (10)
      |
      | *** STATE VARIABLES ***
      | NUM_VARIABLES 4
      | Operative_Level(NUMERIC)(1)(0)
      | TLC_services(NUMERIC_ARRAY)(20)(0  0  0  0  0  0  0  0  0  0  0  0  0  0  0  0  0  0  0  0)
      | Cyber_Fault(NUMERIC_ARRAY)(10)(0  0  0  0  0  0  0  0  0  0)
      | Mechanical_Fault(NUMERIC)(1)(0)
      |
      | *** OUTPUT RESOURCES ***
      | NUM_OUTPUTS 2
      | TLC_SERVICE (20)
      | CYBER_FAULT (10)
      mask step_received=|
      | TLC_services=max(TLC_services_init,TLC_SERVICE);
      | Cyber_Fault=CYBER_FAULT;
      |
      | Operative_Level=min([1-Mechanical_Fault]);
      mask step_sended=|
      | CYBER_FAULT=Cyber_Fault;
      | TLC_SERVICE=TLC_services*Operative_Level;
      mask prompts: Parameter1 "entity name"; Parameter2 "sampling time"; Parameter3 "project"; resources "input resources and state variables"; Parameter10 "Bring state variables to output"; codeupdate "update code from mask"
      mask help: This is a level-2 MATLAB file S-function which demonstrates CISIA entity
      mask DialogControl Container1 Prompt: All parameters
      mask Display: image('Icons/Optical_Switch.png')
  OptSwitch_6 (458) : M-S-Function  FunctionName=cisia_msfun  Parameters=Parameter1, Parameter2, Parameter3, resources, Parameter10, codeupdate, step_received, step_computed, dynamic_computed, step_sended, id_entity, id_project, id_type, name_type, color  mask(S-function:msfcn_unit_delay){Parameter1='OptSwitch_6', Parameter2=1, Parameter3='', resources=|, Parameter10=off, codeupdate=off, step_received=|, step_computed=, dynamic_computed=, step_sended=|, id_entity=458, id_project=6, id_type=102, name_type=Optical_Switch, color=#FFFFFF}
      mask resources=|
      | *** INPUT RESOURCES ***
      | NUM_INPUTS 2
      | TLC_SERVICE (20)
      | CYBER_FAULT (10)
      |
      | *** STATE VARIABLES ***
      | NUM_VARIABLES 4
      | Operative_Level(NUMERIC)(1)(0)
      | TLC_services(NUMERIC_ARRAY)(20)(0  0  0  0  0  0  0  0  0  0  0  0  0  0  0  0  0  0  0  0)
      | Cyber_Fault(NUMERIC_ARRAY)(10)(0  0  0  0  0  0  0  0  0  0)
      | Mechanical_Fault(NUMERIC)(1)(0)
      |
      | *** OUTPUT RESOURCES ***
      | NUM_OUTPUTS 2
      | TLC_SERVICE (20)
      | CYBER_FAULT (10)
      mask step_received=|
      | TLC_services=max(TLC_services_init,TLC_SERVICE);
      | Cyber_Fault=CYBER_FAULT;
      |
      | Operative_Level=min([1-Mechanical_Fault]);
      mask step_sended=|
      | CYBER_FAULT=Cyber_Fault;
      | TLC_SERVICE=TLC_services*Operative_Level;
      mask prompts: Parameter1 "entity name"; Parameter2 "sampling time"; Parameter3 "project"; resources "input resources and state variables"; Parameter10 "Bring state variables to output"; codeupdate "update code from mask"
      mask help: This is a level-2 MATLAB file S-function which demonstrates CISIA entity
      mask DialogControl Container1 Prompt: All parameters
      mask Display: image('Icons/Optical_Switch.png')
  OptSwitch_7 (465) : M-S-Function  FunctionName=cisia_msfun  Parameters=Parameter1, Parameter2, Parameter3, resources, Parameter10, codeupdate, step_received, step_computed, dynamic_computed, step_sended, id_entity, id_project, id_type, name_type, color  mask(S-function:msfcn_unit_delay){Parameter1='OptSwitch_7', Parameter2=1, Parameter3='', resources=|, Parameter10=off, codeupdate=off, step_received=|, step_computed=, dynamic_computed=, step_sended=|, id_entity=465, id_project=6, id_type=102, name_type=Optical_Switch, color=#FFFFFF}
      mask resources=|
      | *** INPUT RESOURCES ***
      | NUM_INPUTS 2
      | TLC_SERVICE (20)
      | CYBER_FAULT (10)
      |
      | *** STATE VARIABLES ***
      | NUM_VARIABLES 4
      | Operative_Level(NUMERIC)(1)(0)
      | TLC_services(NUMERIC_ARRAY)(20)(0  0  0  0  0  0  0  0  0  0  0  0  0  0  0  0  0  0  0  0)
      | Cyber_Fault(NUMERIC_ARRAY)(10)(0  0  0  0  0  0  0  0  0  0)
      | Mechanical_Fault(NUMERIC)(1)(0)
      |
      | *** OUTPUT RESOURCES ***
      | NUM_OUTPUTS 2
      | TLC_SERVICE (20)
      | CYBER_FAULT (10)
      mask step_received=|
      | TLC_services=max(TLC_services_init,TLC_SERVICE);
      | Cyber_Fault=CYBER_FAULT;
      |
      | Operative_Level=min([1-Mechanical_Fault]);
      mask step_sended=|
      | CYBER_FAULT=Cyber_Fault;
      | TLC_SERVICE=TLC_services*Operative_Level;
      mask prompts: Parameter1 "entity name"; Parameter2 "sampling time"; Parameter3 "project"; resources "input resources and state variables"; Parameter10 "Bring state variables to output"; codeupdate "update code from mask"
      mask help: This is a level-2 MATLAB file S-function which demonstrates CISIA entity
      mask DialogControl Container1 Prompt: All parameters
      mask Display: image('Icons/Optical_Switch.png')
  Pipe_3 (345) : M-S-Function  FunctionName=cisia_msfun  Parameters=Parameter1, Parameter2, Parameter3, resources, Parameter10, codeupdate, step_received, step_computed, dynamic_computed, step_sended, id_entity, id_project, id_type, name_type, color  mask(S-function:msfcn_unit_delay){Parameter1='Pipe_3', Parameter2=1, Parameter3='', resources=|, Parameter10=off, codeupdate=off, step_received=|, step_computed=, dynamic_computed=, step_sended=|, id_entity=345, id_project=6, id_type=84, name_type=Pipe, color=#00FFFF}
      mask resources=|
      | *** INPUT RESOURCES ***
      | NUM_INPUTS 3
      | WATER (1)
      | VALVE_QoS (1)
      | PUMP_QoS (1)
      |
      | *** STATE VARIABLES ***
      | NUM_VARIABLES 3
      | Operative_Level(NUMERIC)(1)(1)
      | Mechanical_Fault(NUMERIC)(1)(0)
      | Water_Fault(NUMERIC)(1)(0)
      |
      | *** OUTPUT RESOURCES ***
      | NUM_OUTPUTS 2
      | WATER (1)
      | PIPE_QoS (1)
      mask step_received=|
      | Water_Fault=max([1-WATER Mechanical_Fault 1-VALVE_QoS 1-PUMP_QoS]);
      |
      | Operative_Level=1-Mechanical_Fault;
      mask step_sended=|
      | WATER=1-Water_Fault;
      | PIPE_QoS=Operative_Level;
      mask prompts: Parameter1 "entity name"; Parameter2 "sampling time"; Parameter3 "project"; resources "input resources and state variables"; Parameter10 "Bring state variables to output"; codeupdate "update code from mask"
      mask help: This is a level-2 MATLAB file S-function which demonstrates CISIA entity
      mask DialogControl Container1 Prompt: All parameters
      mask Display: image('Icons/Pipe.png')
  Pipe_5 (347) : M-S-Function  FunctionName=cisia_msfun  Parameters=Parameter1, Parameter2, Parameter3, resources, Parameter10, codeupdate, step_received, step_computed, dynamic_computed, step_sended, id_entity, id_project, id_type, name_type, color  mask(S-function:msfcn_unit_delay){Parameter1='Pipe_5', Parameter2=1, Parameter3='', resources=|, Parameter10=off, codeupdate=off, step_received=|, step_computed=, dynamic_computed=, step_sended=|, id_entity=347, id_project=6, id_type=84, name_type=Pipe, color=#00FFFF}
      mask resources=|
      | *** INPUT RESOURCES ***
      | NUM_INPUTS 3
      | WATER (1)
      | VALVE_QoS (1)
      | PUMP_QoS (1)
      |
      | *** STATE VARIABLES ***
      | NUM_VARIABLES 3
      | Operative_Level(NUMERIC)(1)(1)
      | Mechanical_Fault(NUMERIC)(1)(0)
      | Water_Fault(NUMERIC)(1)(0)
      |
      | *** OUTPUT RESOURCES ***
      | NUM_OUTPUTS 2
      | WATER (1)
      | PIPE_QoS (1)
      mask step_received=|
      | Water_Fault=max([1-WATER Mechanical_Fault 1-VALVE_QoS 1-PUMP_QoS]);
      |
      | Operative_Level=1-Mechanical_Fault;
      mask step_sended=|
      | WATER=1-Water_Fault;
      | PIPE_QoS=Operative_Level;
      mask prompts: Parameter1 "entity name"; Parameter2 "sampling time"; Parameter3 "project"; resources "input resources and state variables"; Parameter10 "Bring state variables to output"; codeupdate "update code from mask"
      mask help: This is a level-2 MATLAB file S-function which demonstrates CISIA entity
      mask DialogControl Container1 Prompt: All parameters
      mask Display: image('Icons/Pipe.png')
  Primary_Cabin_1 (315) : M-S-Function  FunctionName=cisia_msfun  Parameters=Parameter1, Parameter2, Parameter3, resources, Parameter10, codeupdate, step_received, step_computed, dynamic_computed, step_sended, id_entity, id_project, id_type, name_type, color  mask(S-function:msfcn_unit_delay){Parameter1='Primary_Cabin_1', Parameter2=1, Parameter3='', resources=|, Parameter10=off, codeupdate=off, step_received=|, step_computed=, dynamic_computed=, step_sended=E_POWER_1=Power_Gen*(1-Physical_Fault);, id_entity=315, id_project=6, id_type=66, name_type=Electric_Plant, color=#FFFFFF}
      mask resources=|
      | *** INPUT RESOURCES ***
      | NUM_INPUTS 0
      |
      | *** STATE VARIABLES ***
      | NUM_VARIABLES 5
      | Operative_Level(NUMERIC)(1)(1)
      | Mechanical_Fault(NUMERIC)(1)(0)
      | Fire_Fault(NUMERIC)(1)(0)
      | Physical_Fault(NUMERIC)(1)(0)
      | Power_Gen(NUMERIC_ARRAY)(10)(1  0  0  0  0  0  0  0  0  0)
      |
      | *** OUTPUT RESOURCES ***
      | NUM_OUTPUTS 1
      | E_POWER_1 (10)
      mask step_received=|
      | Physical_Fault=max(Fire_Fault,Mechanical_Fault);
      |
      | Operative_Level=1-Physical_Fault;
      mask prompts: Parameter1 "entity name"; Parameter2 "sampling time"; Parameter3 "project"; resources "input resources and state variables"; Parameter10 "Bring state variables to output"; codeupdate "update code from mask"
      mask help: This is a level-2 MATLAB file S-function which demonstrates CISIA entity
      mask DialogControl Container1 Prompt: All parameters
      mask Display: image('Icons/Primary_Cabin_1.png')
  Pump_1 (351) : M-S-Function  FunctionName=cisia_msfun  Parameters=Parameter1, Parameter2, Parameter3, resources, Parameter10, codeupdate, step_received, step_computed, dynamic_computed, step_sended, id_entity, id_project, id_type, name_type, color  mask(S-function:msfcn_unit_delay){Parameter1='Pump_1', Parameter2=1, Parameter3='', resources=|, Parameter10=off, codeupdate=off, step_received=|, step_computed=, dynamic_computed=, step_sended=|, id_entity=351, id_project=6, id_type=85, name_type=Pump, color=#FFFFFF}
      mask resources=|
      | *** INPUT RESOURCES ***
      | NUM_INPUTS 3
      | CYBER_FAULT (10)
      | POWER (1)
      | TELECONTROL (1)
      |
      | *** STATE VARIABLES ***
      | NUM_VARIABLES 14
      | Operative_Level(NUMERIC)(1)(1)
      | Dos_attack(NUMERIC)(1)(0)
      | MITM_attack(NUMERIC)(1)(0)
      | Virus_Attack(NUMERIC)(1)(0)
      | Port_Scan_Attack(NUMERIC)(1)(0)
      | Cyber_Fault(NUMERIC_ARRAY)(10)(0  0  0  0  0  0  0  0  0  0)
      | BGP_hijacking(NUMERIC)(1)(0)
      | Mechanical_Fault(NUMERIC)(1)(0)
      | BotNet_Attack(NUMERIC)(1)(0)
      | Data_Corruption(NUMERIC)(1)(0)
      | SW_Change(NUMERIC)(1)(0)
      | Config_Change(NUMERIC)(1)(0)
      | Port_Saturation(NUMERIC)(1)(0)
      | Control_Fault(NUMERIC)(1)(0)
      |
      | *** OUTPUT RESOURCES ***
      | NUM_OUTPUTS 2
      | CYBER_FAULT (10)
      | PUMP_QoS (1)
      mask step_received=|
      | Cyber_Fault=max(CYBER_FAULT, transpose([Dos_attack MITM_attack Virus_Attack Port_Scan_Attack  BGP_hijacking BotNet_Attack Data_Corruption SW_Change Config_Change Port_Saturation]));
      |
      |
      | Control_Fault=max([1-TELECONTROL Mechanical_Fault Dos_attack min(0.5,max(Cyber_Fault))]);
      |
      |
      | Operative_Level=min([1-Control_Fault 1-max(Cyber_Fault) 1-Mechanical_Fault POWER]);
      mask step_sended=|
      | PUMP_QoS=1-Control_Fault;
      | CYBER_FAULT=Cyber_Fault.*transpose([0 0 0.5 0.2 0 0 0 0 0 0]);
      mask prompts: Parameter1 "entity name"; Parameter2 "sampling time"; Parameter3 "project"; resources "input resources and state variables"; Parameter10 "Bring state variables to output"; codeupdate "update code from mask"
      mask help: This is a level-2 MATLAB file S-function which demonstrates CISIA entity
      mask DialogControl Container1 Prompt: All parameters
      mask Display: image('Icons/Pump.png')
  Residential_1 (337) : M-S-Function  FunctionName=cisia_msfun  Parameters=Parameter1, Parameter2, Parameter3, resources, Parameter10, codeupdate, step_received, step_computed, dynamic_computed, step_sended, id_entity, id_project, id_type, name_type, color  mask(S-function:msfcn_unit_delay){Parameter1='Residential_1', Parameter2=1, Parameter3='', resources=|, Parameter10=off, codeupdate=off, step_received=|, step_computed=, dynamic_computed=, step_sended=RESIDENTIAL_QoS=Operative_Level;, id_entity=337, id_project=6, id_type=89, name_type=Residential, color=#FFFFFF}
      mask resources=|
      | *** INPUT RESOURCES ***
      | NUM_INPUTS 2
      | POWER (1)
      | WATER (1)
      |
      | *** STATE VARIABLES ***
      | NUM_VARIABLES 3
      | Operative_Level(NUMERIC)(1)(1)
      | Power_Fault(NUMERIC)(1)(0)
      | Water_Fault(NUMERIC)(1)(0)
      |
      | *** OUTPUT RESOURCES ***
      | NUM_OUTPUTS 1
      | RESIDENTIAL_QoS (1)
      mask step_received=|
      | Power_Fault=1-POWER;
      | Water_Fault=1-WATER;
      |
      | Operative_Level=min(1-Power_Fault,1-Water_Fault);
      mask prompts: Parameter1 "entity name"; Parameter2 "sampling time"; Parameter3 "project"; resources "input resources and state variables"; Parameter10 "Bring state variables to output"; codeupdate "update code from mask"
      mask help: This is a level-2 MATLAB file S-function which demonstrates CISIA entity
      mask DialogControl Container1 Prompt: All parameters
      mask Display: image('Icons/Residential.png')
  SAVE_2 (2) : M-S-Function  FunctionName=cisia_msfun  Parameters=Parameter1, Parameter2, Parameter3  mask(S-function:msfcn_unit_delay){Parameter1='SAVE_2', Parameter2=1, Parameter3=""}
      mask prompts: Parameter1 "entity name"; Parameter2 "sampling time"; Parameter3 "project"
      mask help: This is a level-2 MATLAB file S-function which demonstrates CISIA entity
      mask Display: disp('SAVE')
  SCADA_1 (442) : M-S-Function  FunctionName=cisia_msfun  Parameters=Parameter1, Parameter2, Parameter3, resources, Parameter10, codeupdate, step_received, step_computed, dynamic_computed, step_sended, id_entity, id_project, id_type, name_type, color  mask(S-function:msfcn_unit_delay){Parameter1='SCADA_1', Parameter2=1, Parameter3='', resources=|, Parameter10=off, codeupdate=off, step_received=|, step_computed=, dynamic_computed=, step_sended=|, id_entity=442, id_project=6, id_type=82, name_type=SCADA, color=#FFFFFF}
      mask resources=|
      | *** INPUT RESOURCES ***
      | NUM_INPUTS 3
      | CYBER_FAULT (10)
      | POWER (1)
      | PLC_QoS (1)
      |
      | *** STATE VARIABLES ***
      | NUM_VARIABLES 14
      | Operative_Level(NUMERIC)(1)(0)
      | Dos_attack(NUMERIC)(1)(0)
      | MITM_attack(NUMERIC)(1)(0)
      | Virus_Attack(NUMERIC)(1)(0)
      | Port_Scan_Attack(NUMERIC)(1)(0)
      | Cyber_Fault(NUMERIC_ARRAY)(10)(0  0  0  0  0  0  0  0  0  0)
      | BGP_hijacking(NUMERIC)(1)(0)
      | Mechanical_Fault(NUMERIC)(1)(0)
      | BotNet_Attack(NUMERIC)(1)(0)
      | Data_Corruption(NUMERIC)(1)(0)
      | SW_Change(NUMERIC)(1)(0)
      | Config_Change(NUMERIC)(1)(0)
      | Port_Saturation(NUMERIC)(1)(0)
      | Control_Fault(NUMERIC)(1)(0)
      |
      | *** OUTPUT RESOURCES ***
      | NUM_OUTPUTS 2
      | CYBER_FAULT (10)
      | SCADA_QoS (1)
      mask step_received=|
      | Cyber_Fault=max(CYBER_FAULT, transpose([Dos_attack MITM_attack Virus_Attack Port_Scan_Attack  BGP_hijacking BotNet_Attack Data_Corruption SW_Change Config_Change Port_Saturation]));
      |
      |
      | Control_Fault=max([Mechanical_Fault Dos_attack min(0.5,max(Cyber_Fault))]);
      |
      |
      |
      | Operative_Level=min([1-max(Cyber_Fault) 1-Mechanical_Fault POWER PLC_QoS]);
      mask step_sended=|
      | SCADA_QoS=Operative_Level;
      |
      | CYBER_FAULT=Cyber_Fault.*transpose([0 0 0.5 0.2 0 0 0 0 0 0]);
      mask prompts: Parameter1 "entity name"; Parameter2 "sampling time"; Parameter3 "project"; resources "input resources and state variables"; Parameter10 "Bring state variables to output"; codeupdate "update code from mask"
      mask help: This is a level-2 MATLAB file S-function which demonstrates CISIA entity
      mask DialogControl Container1 Prompt: All parameters
      mask Display: image('Icons/SCADA.png')
  Scope : Scope
  Solar_1 (453) : M-S-Function  FunctionName=cisia_msfun  Parameters=Parameter1, Parameter2, Parameter3, resources, Parameter10, codeupdate, step_received, step_computed, dynamic_computed, step_sended, id_entity, id_project, id_type, name_type, color  mask(S-function:msfcn_unit_delay){Parameter1='Solar_1', Parameter2=1, Parameter3='', resources=|, Parameter10=off, codeupdate=off, step_received=|, step_computed=, dynamic_computed=, step_sended=IoT_measure=(1-IoT_Fault)*Operative_Level;, id_entity=453, id_project=6, id_type=104, name_type=Solar_Panels, color=#FFFFFF}
      mask resources=|
      | *** INPUT RESOURCES ***
      | NUM_INPUTS 1
      | TELECONTROL (1)
      |
      | *** STATE VARIABLES ***
      | NUM_VARIABLES 5
      | Operative_Level(NUMERIC)(1)(1)
      | Mechanical_Fault(NUMERIC)(1)(0)
      | Consumed_Services(NUMERIC_ARRAY)(20)(1  0  0  0  0  0  0  0  0  0  0  0  0  0  0  0  0  0  0  0)
      | Control_Fault(NUMERIC)(1)(0)
      | IoT_Fault(NUMERIC)(1)(0)
      |
      | *** OUTPUT RESOURCES ***
      | NUM_OUTPUTS 1
      | IoT_measure (1)
      mask step_received=|
      | Control_Fault=max([1-TELECONTROL Mechanical_Fault]);
      |
      | Operative_Level=min([1- Control_Fault 1-Mechanical_Fault]);
      mask prompts: Parameter1 "entity name"; Parameter2 "sampling time"; Parameter3 "project"; resources "input resources and state variables"; Parameter10 "Bring state variables to output"; codeupdate "update code from mask"
      mask help: This is a level-2 MATLAB file S-function which demonstrates CISIA entity
      mask DialogControl Container1 Prompt: All parameters
      mask Display: image('Icons/Solar_Panels.png')
  Substation_1 (441) : M-S-Function  FunctionName=cisia_msfun  Parameters=Parameter1, Parameter2, Parameter3, resources, Parameter10, codeupdate, step_received, step_computed, dynamic_computed, step_sended, id_entity, id_project, id_type, name_type, color  mask(S-function:msfcn_unit_delay){Parameter1='Substation_1', Parameter2=1, Parameter3='', resources=|, Parameter10=off, codeupdate=off, step_received=|, step_computed=, dynamic_computed=, step_sended=POWER=Operative_Level;, id_entity=441, id_project=6, id_type=100, name_type=SecondarySubstation, color=#FFFFFF}
      mask resources=|
      | *** INPUT RESOURCES ***
      | NUM_INPUTS 1
      | E_POWER_1 (10)
      |
      | *** STATE VARIABLES ***
      | NUM_VARIABLES 4
      | Operative_Level(NUMERIC)(1)(1)
      | Mechanical_Fault(NUMERIC)(1)(0)
      | Power_Fault(NUMERIC)(1)(0)
      | Consumed_Power(NUMERIC_ARRAY)(10)(1  0  0  0  0  0  0  0  0  0)
      |
      | *** OUTPUT RESOURCES ***
      | NUM_OUTPUTS 1
      | POWER (1)
      mask step_received=|
      | Power_Fault=max(abs(Consumed_Power.*E_POWER_1-Consumed_Power));
      |
      |
      | Operative_Level=max([1-Power_Fault 0.5])*(1-Mechanical_Fault);
      mask prompts: Parameter1 "entity name"; Parameter2 "sampling time"; Parameter3 "project"; resources "input resources and state variables"; Parameter10 "Bring state variables to output"; codeupdate "update code from mask"
      mask help: This is a level-2 MATLAB file S-function which demonstrates CISIA entity
      mask DialogControl Container1 Prompt: All parameters
      mask Display: image('Icons/SecondarySubstation.png')
  Tank_1 (334) : M-S-Function  FunctionName=cisia_msfun  Parameters=Parameter1, Parameter2, Parameter3, resources, Parameter10, codeupdate, step_received, step_computed, dynamic_computed, step_sended, id_entity, id_project, id_type, name_type, color  mask(S-function:msfcn_unit_delay){Parameter1='Tank_1', Parameter2=1, Parameter3='', resources=|, Parameter10=off, codeupdate=off, step_received=|, step_computed=Water_Level_new=max(0,Water_Level-0.2*Water_Fault);, dynamic_computed=, step_sended=|, id_entity=334, id_project=6, id_type=87, name_type=Tank, color=#FFFFFF}
      mask resources=|
      | *** INPUT RESOURCES ***
      | NUM_INPUTS 2
      | CYBER_FAULT (10)
      | WATER (1)
      |
      | *** STATE VARIABLES ***
      | NUM_VARIABLES 16
      | Operative_Level(NUMERIC)(1)(1)
      | Dos_attack(NUMERIC)(1)(0)
      | MITM_attack(NUMERIC)(1)(0)
      | Virus_Attack(NUMERIC)(1)(0)
      | Port_Scan_Attack(NUMERIC)(1)(0)
      | Cyber_Fault(NUMERIC_ARRAY)(10)(0  0  0  0  0  0  0  0  0  0)
      | BGP_hijacking(NUMERIC)(1)(0)
      | Mechanical_Fault(NUMERIC)(1)(0)
      | BotNet_Attack(NUMERIC)(1)(0)
      | Data_Corruption(NUMERIC)(1)(0)
      | SW_Change(NUMERIC)(1)(0)
      | Config_Change(NUMERIC)(1)(0)
      | Port_Saturation(NUMERIC)(1)(0)
      | Water_Fault(NUMERIC)(1)(0)
      | Water_Level(NUMERIC)(1)(1)
      | IoT_Fault(NUMERIC)(1)(0)
      |
      | *** OUTPUT RESOURCES ***
      | NUM_OUTPUTS 3
      | CYBER_FAULT (10)
      | WATER (1)
      | IoT_measure (1)
      mask step_received=|
      | Cyber_Fault=max(CYBER_FAULT, transpose([Dos_attack MITM_attack Virus_Attack Port_Scan_Attack  BGP_hijacking BotNet_Attack Data_Corruption SW_Change Config_Change Port_Saturation]));
      |
      | Water_Fault=1-WATER;
      |
      | Operative_Level=min([1-max(Cyber_Fault) 1-Mechanical_Fault 1-IoT_Fault]);
      mask step_sended=|
      | WATER=Water_Level*Operative_Level;
      |
      | CYBER_FAULT=Cyber_Fault.*transpose([0 0 0.5 0.2 0 0 0 0 0 0]);
      |
      | IoT_measure=min([1-IoT_Fault  1-max(Cyber_Fault)]);
      mask prompts: Parameter1 "entity name"; Parameter2 "sampling time"; Parameter3 "project"; resources "input resources and state variables"; Parameter10 "Bring state variables to output"; codeupdate "update code from mask"
      mask help: This is a level-2 MATLAB file S-function which demonstrates CISIA entity
      mask DialogControl Container1 Prompt: All parameters
      mask Display: image('Icons/Tank.png')
  Valve_1 (340) : M-S-Function  FunctionName=cisia_msfun  Parameters=Parameter1, Parameter2, Parameter3, resources, Parameter10, codeupdate, step_received, step_computed, dynamic_computed, step_sended, id_entity, id_project, id_type, name_type, color  mask(S-function:msfcn_unit_delay){Parameter1='Valve_1', Parameter2=1, Parameter3='', resources=|, Parameter10=off, codeupdate=off, step_received=|, step_computed=, dynamic_computed=, step_sended=|, id_entity=340, id_project=6, id_type=86, name_type=Valve, color=#FFFFFF}
      mask resources=|
      | *** INPUT RESOURCES ***
      | NUM_INPUTS 3
      | CYBER_FAULT (10)
      | POWER (1)
      | TELECONTROL (1)
      |
      | *** STATE VARIABLES ***
      | NUM_VARIABLES 16
      | Operative_Level(NUMERIC)(1)(1)
      | Dos_attack(NUMERIC)(1)(0)
      | MITM_attack(NUMERIC)(1)(0)
      | Virus_Attack(NUMERIC)(1)(0)
      | Port_Scan_Attack(NUMERIC)(1)(0)
      | Cyber_Fault(NUMERIC_ARRAY)(10)(0  0  0  0  0  0  0  0  0  0)
      | BGP_hijacking(NUMERIC)(1)(0)
      | Mechanical_Fault(NUMERIC)(1)(0)
      | Unauthorized_Access(NUMERIC)(1)(0)
      | BotNet_Attack(NUMERIC)(1)(0)
      | Data_Corruption(NUMERIC)(1)(0)
      | Rouge_Access(NUMERIC)(1)(0)
      | SW_Change(NUMERIC)(1)(0)
      | Config_Change(NUMERIC)(1)(0)
      | Port_Saturation(NUMERIC)(1)(0)
      | Control_Fault(NUMERIC)(1)(0)
      |
      | *** OUTPUT RESOURCES ***
      | NUM_OUTPUTS 2
      | CYBER_FAULT (10)
      | VALVE_QoS (1)
      mask step_received=|
      | Cyber_Fault=max(CYBER_FAULT, transpose([Dos_attack MITM_attack Virus_Attack Port_Scan_Attack  BGP_hijacking BotNet_Attack Data_Corruption SW_Change Config_Change Port_Saturation]));
      |
      |
      | Control_Fault=max([1-TELECONTROL Mechanical_Fault Dos_attack min(0.5,max(Cyber_Fault))]);
      |
      |
      |
      | Operative_Level=min([1-max(Cyber_Fault) 1-Mechanical_Fault POWER]);
      mask step_sended=|
      | VALVE_QoS=Operative_Level;
      |
      | CYBER_FAULT=Cyber_Fault.*transpose([0 0 0.5 0.2 0 0 0 0 0 0]);
      mask prompts: Parameter1 "entity name"; Parameter2 "sampling time"; Parameter3 "project"; resources "input resources and state variables"; Parameter10 "Bring state variables to output"; codeupdate "update code from mask"
      mask help: This is a level-2 MATLAB file S-function which demonstrates CISIA entity
      mask DialogControl Container1 Prompt: All parameters
      mask Display: image('Icons/Valve.png')
  Water_Controller (466) : M-S-Function  FunctionName=cisia_msfun  Parameters=Parameter1, Parameter2, Parameter3, resources, Parameter10, codeupdate, step_received, step_computed, dynamic_computed, step_sended, id_entity, id_project, id_type, name_type, color  mask(S-function:msfcn_unit_delay){Parameter1='Water_Controller', Parameter2=1, Parameter3='', resources=|, Parameter10=off, codeupdate=off, step_received=|, step_computed=, dynamic_computed=, step_sended=TLC_SERVICE=TLC_services*(1-Mechanical_Fault);, id_entity=466, id_project=6, id_type=103, name_type=Intelligent_Controller, color=#FFFFFF}
      mask resources=|
      | *** INPUT RESOURCES ***
      | NUM_INPUTS 2
      | TLC_SERVICE (20)
      | SCADA_QoS (1)
      |
      | *** STATE VARIABLES ***
      | NUM_VARIABLES 5
      | Operative_Level(NUMERIC)(1)(0)
      | TLC_services(NUMERIC_ARRAY)(20)(0  0  0  0  0  0  1  0  0  0  0  0  0  0  0  0  0  0  0  0)
      | Mechanical_Fault(NUMERIC)(1)(0.6)
      | Consumed_Services(NUMERIC_ARRAY)(20)(0  0  0  0  0  0  0  0  0  0  0  0  0  0  0  0  0  0  0  0)
      | Service_Fault(NUMERIC)(1)(0)
      |
      | *** OUTPUT RESOURCES ***
      | NUM_OUTPUTS 1
      | TLC_SERVICE (20)
      mask step_received=|
      | TLC_services=max(TLC_services_init,TLC_SERVICE);
      |
      | Service_Fault=max(abs(Consumed_Services.*TLC_services-Consumed_Services));
      |
      | Operative_Level=min([1-Mechanical_Fault 1-Service_Fault]);
      mask prompts: Parameter1 "entity name"; Parameter2 "sampling time"; Parameter3 "project"; resources "input resources and state variables"; Parameter10 "Bring state variables to output"; codeupdate "update code from mask"
      mask help: This is a level-2 MATLAB file S-function which demonstrates CISIA entity
      mask DialogControl Container1 Prompt: All parameters
      mask Display: image('Icons/Intelligent_Controller.png')
  Wind_1 (455) : M-S-Function  FunctionName=cisia_msfun  Parameters=Parameter1, Parameter2, Parameter3, resources, Parameter10, codeupdate, step_received, step_computed, dynamic_computed, step_sended, id_entity, id_project, id_type, name_type, color  mask(S-function:msfcn_unit_delay){Parameter1='Wind_1', Parameter2=1, Parameter3='', resources=|, Parameter10=off, codeupdate=off, step_received=|, step_computed=, dynamic_computed=, step_sended=IoT_measure=(1-IoT_Fault)*Operative_Level;, id_entity=455, id_project=6, id_type=106, name_type=WindFarm, color=#FFFFFF}
      mask resources=|
      | *** INPUT RESOURCES ***
      | NUM_INPUTS 1
      | TELECONTROL (1)
      |
      | *** STATE VARIABLES ***
      | NUM_VARIABLES 5
      | Operative_Level(NUMERIC)(1)(1)
      | Mechanical_Fault(NUMERIC)(1)(0)
      | Consumed_Services(NUMERIC_ARRAY)(20)(1  0  0  0  0  0  0  0  0  0  0  0  0  0  0  0  0  0  0  0)
      | Control_Fault(NUMERIC)(1)(0)
      | IoT_Fault(NUMERIC)(1)(0)
      |
      | *** OUTPUT RESOURCES ***
      | NUM_OUTPUTS 1
      | IoT_measure (1)
      mask step_received=|
      | Control_Fault=max([1-TELECONTROL Mechanical_Fault]);
      |
      | Operative_Level=min([1- Control_Fault 1-Mechanical_Fault]);
      mask prompts: Parameter1 "entity name"; Parameter2 "sampling time"; Parameter3 "project"; resources "input resources and state variables"; Parameter10 "Bring state variables to output"; codeupdate "update code from mask"
      mask help: This is a level-2 MATLAB file S-function which demonstrates CISIA entity
      mask DialogControl Container1 Prompt: All parameters
      mask Display: image('Icons/WindFarm.png')
  wires:
  E_Pole_1 (311)/1 -> E_Wire_2 (308)/2  "E_POWER_1"
  Ground2/1 -> E_Wire_1 (307)/1  "FLAME"
  E_Wire_2 (308)/2 -> E_Pole_1 (311)/3  "E_POWER_2"
  E_Wire_1 (307)/1 -> E_Pole_1 (311)/2  "E_POWER_1"
  E_Pole_1 (311)/2 -> E_Wire_1 (307)/3  "E_POWER_2"
  Primary_Cabin_1 (315)/1 -> E_Wire_1 (307)/2  "E_POWER_1"
  Mux2/1 -> Display/1, Mean1/1
  Mean1/1 -> SAVE_2 (2)/1  "SERVICES_QoS"
  CISIA_MASTER (0)/1 -> Display18/1  "MINOR HITS"
  CISIA_MASTER (0)/2 -> Display19/1  "MAJOR HITS"
  CISIA_MASTER (0)/4 -> Display21/1  "TIME PAST"
  CISIA_MASTER (0)/3 -> Display20/1  "DELTA TIME"
  E_Wire_2 (308)/1 -> Substation_1 (441)/1  "E_POWER_1"
  Ground1/1 -> E_Wire_2 (308)/1  "FLAME"
  Ground3/1 -> E_Wire_2 (308)/3  "E_POWER_2"
  Ground4/1 -> E_Pole_1 (311)/1  "FLAME"
  SCADA_1 (442)/2 -> Water_Controller (466)/2, Load_Balancing_1 (446)/2, [SCADA_QoS]  "SCADA_QoS"
  Local_PLC_1 (459)/1 -> MinMax7/1  "TLC_SERVICE"
  MinMax1/1 -> OptSwitch_2 (447)/2  "CYBER_FAULT"
  SCADA_1 (442)/1 -> MinMax1/1, MinMax2/1, MinMax3/1, MinMax13/1, MinMax6/1, MinMax4/1  "CYBER_FAULT"
  OptSwitch_2 (447)/2 -> Local_PLC_1 (459)/2  "CYBER_FAULT"
  E_STORAGE_1 (443)/1 -> Local_PLC_1 (459)/4  "IoT_measure"
  OptSwitch_1 (445)/2 -> SCADA_1 (442)/1  "CYBER_FAULT"
  OptSwitch_1 (445)/1 -> MinMax10/2, MinMax11/2, MinMax14/2, MinMax8/2, MinMax9/2, MinMax7/2, Water_Controller (466)/1, Load_Balancing_1 (446)/1  "TLC_SERVICE"
  OptSwitch_3 (448)/2 -> Local_PLC_2 (460)/2  "CYBER_FAULT"
  OptSwitch_4 (449)/2 -> Local_PLC_3 (461)/2  "CYBER_FAULT"
  OptSwitch_5 (450)/2 -> Local_PLC_4 (462)/2  "CYBER_FAULT"
  MinMax2/1 -> OptSwitch_3 (448)/2  "CYBER_FAULT"
  MinMax3/1 -> OptSwitch_4 (449)/2  "CYBER_FAULT"
  MinMax4/1 -> OptSwitch_5 (450)/2  "CYBER_FAULT"
  MinMax5/1 -> SCADA_1 (442)/3  "PLC_QoS"
  [SCADA_QoS] -> Mux2/1
  MinMax/1 -> OptSwitch_1 (445)/2  "CYBER_FAULT"
  MinMax6/1 -> OptSwitch_6 (458)/2  "CYBER_FAULT"
  OptSwitch_6 (458)/2 -> Local_PLC_5 (463)/2  "CYBER_FAULT"
  Geo_1 (456)/1 -> Local_PLC_5 (463)/4  "IoT_measure"
  OptSwitch_2 (447)/1 -> MinMax12/1, Local_PLC_1 (459)/1  "TLC_SERVICE"
  OptSwitch_3 (448)/1 -> MinMax12/2, Local_PLC_2 (460)/1  "TLC_SERVICE"
  OptSwitch_4 (449)/1 -> Local_PLC_3 (461)/1, MinMax12/3  "TLC_SERVICE"
  OptSwitch_5 (450)/1 -> MinMax12/4, Local_PLC_4 (462)/1  "TLC_SERVICE"
  OptSwitch_6 (458)/1 -> MinMax12/5, Local_PLC_5 (463)/1  "TLC_SERVICE"
  Local_PLC_1 (459)/2 -> MinMax/1, MinMax1/2  "CYBER_FAULT"
  Wind_1 (455)/1 -> Local_PLC_4 (462)/4  "IoT_measure"
  Hydro_1 (454)/1 -> Local_PLC_3 (461)/4  "IoT_measure"
  Solar_1 (453)/1 -> Local_PLC_2 (460)/4  "IoT_measure"
  MinMax7/1 -> OptSwitch_2 (447)/1  "TLC_SERVICE"
  Local_PLC_1 (459)/3 -> E_STORAGE_1 (443)/2  "TELECONTROL"
  Local_PLC_2 (460)/3 -> Solar_1 (453)/1  "TELECONTROL"
  Local_PLC_3 (461)/3 -> Hydro_1 (454)/1  "TELECONTROL"
  Local_PLC_4 (462)/3 -> Wind_1 (455)/1  "TELECONTROL"
  Local_PLC_5 (463)/3 -> Geo_1 (456)/1  "TELECONTROL"
  Local_PLC_1 (459)/4 -> MinMax5/1  "PLC_QoS"
  Local_PLC_2 (460)/4 -> MinMax5/2  "PLC_QoS"
  Local_PLC_3 (461)/4 -> MinMax5/3  "PLC_QoS"
  Local_PLC_4 (462)/4 -> MinMax5/4  "PLC_QoS"
  Local_PLC_5 (463)/4 -> MinMax5/5  "PLC_QoS"
  MinMax8/1 -> OptSwitch_6 (458)/1  "TLC_SERVICE"
  Local_PLC_5 (463)/1 -> MinMax8/1  "TLC_SERVICE"
  MinMax10/1 -> OptSwitch_4 (449)/1  "TLC_SERVICE"
  MinMax9/1 -> OptSwitch_3 (448)/1  "TLC_SERVICE"
  MinMax11/1 -> OptSwitch_5 (450)/1  "TLC_SERVICE"
  Local_PLC_2 (460)/1 -> MinMax9/1  "TLC_SERVICE"
  Local_PLC_3 (461)/1 -> MinMax10/1  "TLC_SERVICE"
  Local_PLC_4 (462)/1 -> MinMax11/1  "TLC_SERVICE"
  Local_PLC_2 (460)/2 -> MinMax/2, MinMax2/2  "CYBER_FAULT"
  Local_PLC_5 (463)/2 -> MinMax/5, MinMax6/2  "CYBER_FAULT"
  Local_PLC_4 (462)/2 -> MinMax/4, MinMax4/2  "CYBER_FAULT"
  Local_PLC_3 (461)/2 -> MinMax/3, MinMax3/2  "CYBER_FAULT"
  MinMax12/1 -> OptSwitch_1 (445)/1  "TLC_SERVICE"
  Load_Balancing_1 (446)/1 -> MinMax12/6  "TLC_SERVICE"
  Substation_1 (441)/1 -> E_STORAGE_1 (443)/1, SCADA_1 (442)/2, Local_PLC_1 (459)/3, Local_PLC_2 (460)/3, Local_PLC_3 (461)/3, Residential_1 (337)/1, Valve_1 (340)/2, Pump_1 (351)/2, Local_PLC_6 (464)/3, Local_PLC_5 (463)/3, Local_PLC_4 (462)/3  "POWER"
  Residential_1 (337)/1 -> [RESIDENTIAL_1_QoS]  "RESIDENTIAL_QoS"
  Pipe_3 (345)/1 -> Residential_1 (337)/2  "WATER"
  Constant2/1 -> Pipe_3 (345)/3  "PUMP_QoS"
  Constant4/1 -> Pipe_5 (347)/2  "VALVE_QoS"
  Pipe_5 (347)/1 -> Tank_1 (334)/2  "WATER"
  Pump_1 (351)/2 -> Scope/1, Pipe_5 (347)/3  "PUMP_QoS"
  Tank_1 (334)/2 -> [Water_Tank], Pipe_3 (345)/1  "WATER"
  Valve_1 (340)/2 -> Pipe_3 (345)/2  "VALVE_QoS"
  Constant1/1 -> Pipe_5 (347)/1  "WATER"
  Tank_1 (334)/3 -> Local_PLC_6 (464)/4  "IoT_measure"
  Local_PLC_6 (464)/3 -> Valve_1 (340)/3, Pump_1 (351)/3  "TELECONTROL"
  OptSwitch_7 (465)/2 -> Local_PLC_6 (464)/2  "CYBER_FAULT"
  MinMax13/1 -> OptSwitch_7 (465)/2  "CYBER_FAULT"
  OptSwitch_7 (465)/1 -> Local_PLC_6 (464)/1  "TLC_SERVICE"
  Local_PLC_6 (464)/1 -> MinMax14/1  "TLC_SERVICE"
  MinMax14/1 -> OptSwitch_7 (465)/1  "TLC_SERVICE"
  Local_PLC_6 (464)/2 -> Pump_1 (351)/1, Valve_1 (340)/1, Tank_1 (334)/1, MinMax13/2  "CYBER_FAULT"
  Water_Controller (466)/1 -> MinMax12/7  "TLC_SERVICE"
  [RESIDENTIAL_1_QoS] -> Mux2/2
  [RESIDENTIAL_1_QoS] -> Mux2/3
